simulink subsystem "MPC11_nlpsol"  (R2022b)
settings: Solver=VariableStepAuto  StartTime=0.0  StopTime=10.0  RelTol=1e-3
undefined symbols (not defined in the file): param_MPC11, param_traj_data, param_weight_init
settings Model: Creator=emu  LastModifiedBy=emu
settings OptimizationCC: ReuseModelBlockBuffer=on

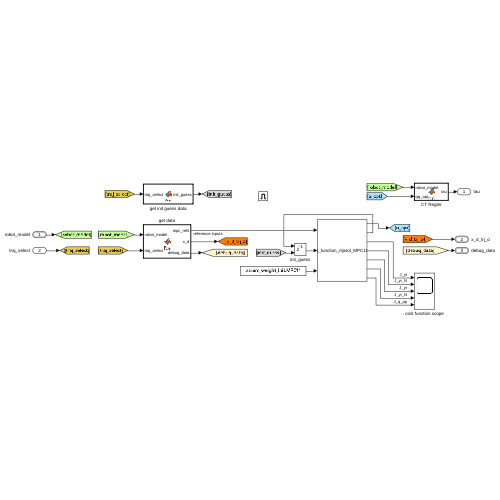
[thumbnail: Simulink's stored preview of the top-level diagram]
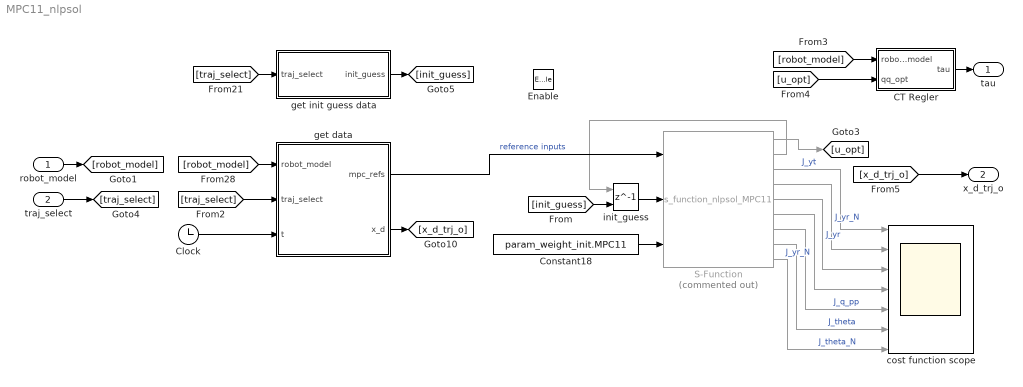
== system MPC11_nlpsol ==
  robot_model : Inport  OutDataTypeStr=Bus: robot_model
  traj_select : Inport  Port=2
  Enable : EnablePort
  CT Regler : MATLAB Function  TreatAsAtomicUnit=on
  Clock : Clock
  Constant18 : Constant  Value=param_weight_init.MPC11  VectorParams1D=off
  S-Function : S-Function  Commented=on  FunctionName=s_function_nlpsol_MPC11  Parameters='s_functions/ur5e_6dof/MPC11.casadi', 'MPC11'  SFunctionModules='MPC11'  SFunctionDeploymentMode=off  EnableBusSupport=off
  cost function scope : Scope  NumInputPorts=7
  get data : MATLAB Function  TreatAsAtomicUnit=on
  get init guess data : MATLAB Function  TreatAsAtomicUnit=on
  init_guess : Delay  DelayLength=1  InitialConditionSource=Input port  InitialCondition=1
      settings: InputPortMap=u0,p4
  tau : Outport
  x_d_trj_o : Outport  Port=2  OutDataTypeStr=Bus: x_d
  wires:
  S-Function/2 -> init_guess/1
  S-Function/7 -> cost function scope/5  "J_q_pp"
  get data/1(mpc_refs) -> S-Function/1  "reference inputs"
  [robot_model] -> get data/1(robot_model)
  get data/2(x_d) -> [x_d_trj_o]
  [traj_select] -> get init guess data/1(traj_select)
  [init_guess] -> init_guess/2
  CT Regler/1(tau) -> tau/1
  S-Function/6 -> cost function scope/4  "J_yr_N"
  traj_select/1 -> [traj_select]
  [u_opt] -> CT Regler/2(qq_opt)
  S-Function/4 -> cost function scope/2  "J_yr_N"
  [traj_select] -> get data/2(traj_select)
  [robot_model] -> CT Regler/1(robot_model)
  robot_model/1 -> [robot_model]
  init_guess/1 -> S-Function/2
  get init guess data/1(init_guess) -> [init_guess]
  Constant18/1 -> S-Function/3
  S-Function/3 -> cost function scope/1  "J_yt"
  S-Function/5 -> cost function scope/3  "J_yr"
  [x_d_trj_o] -> x_d_trj_o/1
  S-Function/1 -> [u_opt]
  Clock/1 -> get data/3(t)
  S-Function/8 -> cost function scope/6  "J_theta"
  S-Function/9 -> cost function scope/7  "J_theta_N"

== matlab function MPC11_nlpsol/CT Regler ==
  data: robot_model input Bus: robot_model; tau output; qq_opt input
function tau = fcn(robot_model, qq_opt)

if size(qq_opt, 2) ~= 0 && size(qq_opt, 1) ~= 1
    q_d_pp = qq_opt;

    M = robot_model.M;      % inertia matrix
    C_rnea = robot_model.C_rnea; % C_rnea(q, q_p) = C(q, q_p)q_p + g(q) = n(q, q_p)
    
    tau = M*q_d_pp + C_rnea;
else
    tau = zeros(6,1);
end

== matlab function MPC11_nlpsol/get data ==
  settings: updateMethod=DISCRETE  sampleTime=param_global.Ta
  data: mpc_refs output; robot_model input Bus: robot_model; param_MPC11 parameter; x_d output Bus: x_d; param_traj_data parameter; traj_select input; t input
function [mpc_refs, x_d] = fcn(robot_model, param_MPC11, param_traj_data, traj_select, t)
persistent cnt;

if(isempty(cnt))
    cnt = 1;
end

param_MPC = param_MPC11;
N         = param_MPC.N;
N_step    = param_MPC.N_step;

% Parameters
q    = robot_model.q;      % generalized coordinates
q_p  = robot_model.q_p;  % time derivative of generalized coordinates

x_k = [q;q_p];

% Assemble vector of recieved output measurements
p_d    = param_traj_data.p_d(   1:3, cnt : N_step : cnt + (N)*N_step, traj_select);
%p_d_p  = param_traj_data.p_d_p( 1:3, cnt : N_step : cnt + (N)*N_step, traj_select);
%p_d_pp = param_traj_data.p_d_pp(1:3, cnt : N_step : cnt + (N)*N_step, traj_select);

% RPY XYZ angles
%Phi_d = param_traj_data.Phi_d(      1:3, cnt : N_step : cnt + (N) * N_step, traj_select ); % (Phi_0 ... Phi_N)
%Phi_d_p = param_traj_data.Phi_d_p(  1:3, cnt : N_step : cnt + (N) * N_step, traj_select ); % (Phi_p_0 ... Phi_p_N)
%Phi_d_pp = param_traj_data.Phi_d_pp(1:3, cnt : N_step : cnt + (N) * N_step, traj_select ); % (Phi_pp_0 ... Phi_pp_N)

q_d    = param_traj_data.q_d(      1:4, cnt : N_step : cnt + (N)*N_step, traj_select);
%q_d_p  = param_traj_data.q_d_p(    1:4, cnt : N_step : cnt + (N)*N_step, traj_select);
%q_d_pp = param_traj_data.q_d_pp(   1:4, cnt : N_step : cnt + (N)*N_step, traj_select);

omega_d   = param_traj_data.omega_d(  1:3, cnt : N_step : cnt + (N)*N_step, traj_select);
omega_d_p = param_traj_data.omega_d_p(1:3, cnt : N_step : cnt + (N)*N_step, traj_select);

alpha_d    = param_traj_data.alpha_d(           :, cnt : N_step : cnt + (N)*N_step, traj_select);
alpha_d_p  = param_traj_data.alpha_d_p(         :, cnt : N_step : cnt + (N)*N_step, traj_select);
alpha_d_pp = param_traj_data.alpha_d_pp(        :, cnt : N_step : cnt + (N)*N_step, traj_select);
rot_ax_d   = param_traj_data.rot_ax_d(          :, cnt : N_step : cnt + (N)*N_step, traj_select);
alpha_d_offset = param_traj_data.alpha_d_offset(:, cnt : N_step : cnt + (N)*N_step, traj_select);
q_d_rel = param_traj_data.q_d_rel(              :, cnt : N_step : cnt + (N)*N_step, traj_select);

%y_d = [p_d; q_d];
%y_d_p = [p_d_p; omega_d];
%y_d_pp = [p_d_pp; omega_d_p];

%% Reference out
mpc_refs = [x_k(:); t];

%% TRAJECTORY OUT
x_d.p_d       = param_traj_data.p_d(1:3, cnt , traj_select);    %y0
x_d.p_d_p     = param_traj_data.p_d_p(1:3, cnt , traj_select);  %y0p
x_d.p_d_pp    = param_traj_data.p_d_pp(1:3, cnt , traj_select); %y0pp
x_d.Phi_d     = param_traj_data.Phi_d(:, cnt , traj_select);
x_d.Phi_d_p   = param_traj_data.Phi_d_p(:, cnt, traj_select);
x_d.Phi_d_pp  = param_traj_data.Phi_d_pp(:,cnt, traj_select);
x_d.R_d       = param_traj_data.R_d(:,:, cnt, traj_select);
x_d.q_d       = q_d(1:4, 1);
x_d.q_d_p     = param_traj_data.q_d_p(1:4, cnt, traj_select);
x_d.q_d_pp    = param_traj_data.q_d_pp(1:4, cnt, traj_select);
x_d.omega_d   = omega_d(1:3, 1);
x_d.omega_d_p = omega_d_p(1:3, 1);
x_d.alpha_d    = alpha_d(:, 1);
x_d.alpha_d_p  = alpha_d_p(:, 1);
x_d.alpha_d_pp = alpha_d_pp(:, 1);
x_d.rot_ax_d   = rot_ax_d(:, 1);
x_d.alpha_d_offset = alpha_d_offset(:, 1);
x_d.q_d_rel = q_d_rel(:, 1);

cnt = cnt+1;

== matlab function MPC11_nlpsol/get init guess data ==
  data: traj_select input; param_MPC11_init_guess parameter; init_guess output
function init_guess   = fcn(traj_select, param_MPC11_init_guess)

%init_guess = param_MPC11_init_guess.init_guess(1,:);
init_guess = param_MPC11_init_guess.init_guess(traj_select,:);
